simulink model "fullsys_version"  (R2022b)
settings: Solver=VariableStepAuto  StartTime=0.0  StopTime=13  RelTol=1e-3
values from neighbouring files (symbols this model uses):
  alpha_trim = (((Cz_trim + Cz_alp*alpha_0)*(-1*Cm_delm)/Cz_delm) - Cm_0 + (alpha_0*Cm_alpha))/(Cm_alpha + (Cz_alp*(-1*Cm_delm)/Cz_delm))    [variableLoader.m]    (also in variableLoader_OLD.m)
  delt_trim = double(Vin_trim/44.4)    [variableLoader.m]    (also in variableLoader_OLD.m = sqrt((T_trim/(ro*Sprop*Cprop/(2*m))) + velocity*velocity)/kM)
  delta_m_trim = ((alpha_trim - alpha_0)*Cm_alpha + Cm_0)/(-1*Cm_delm)    [variableLoader.m]    (also in variableLoader_OLD.m)
  velocity = 25    [variableLoader.m]    (also in variableLoader_OLD.m)

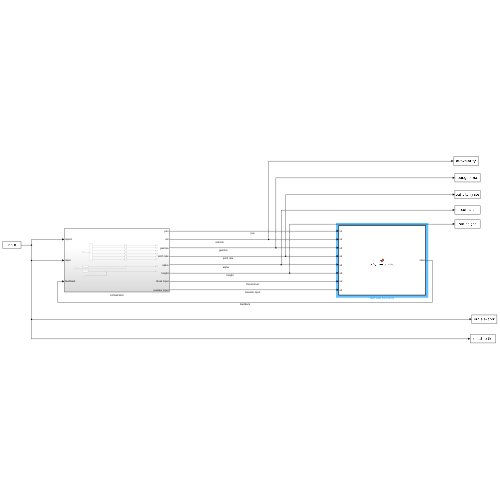
[thumbnail: Simulink's stored preview of the top-level diagram]
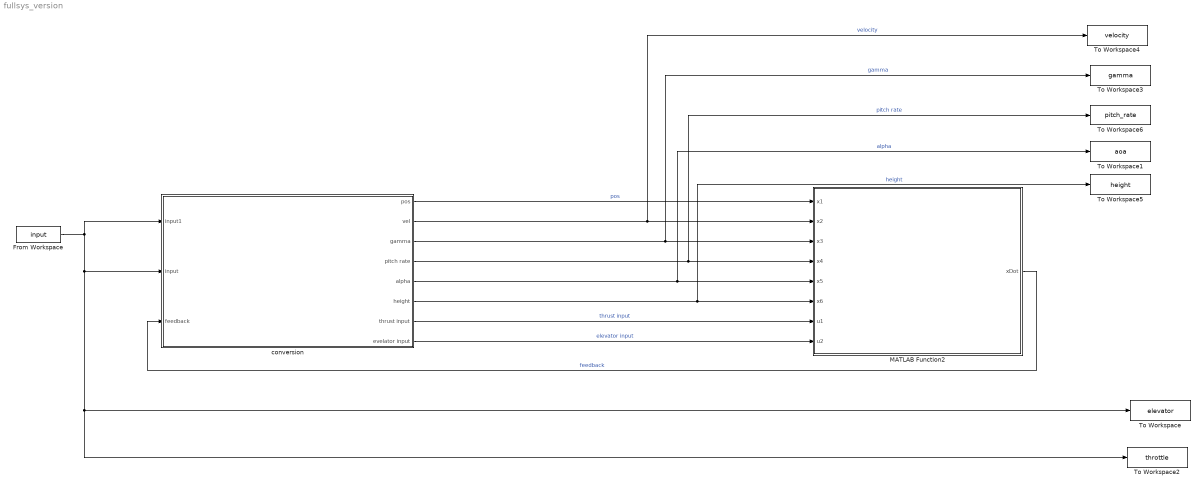
== system fullsys_version ==
  From Workspace : FromWorkspace  VariableName=input  SampleTime=0.02
  MATLAB Function2 : MATLAB Function  TreatAsAtomicUnit=on
  To Workspace : ToWorkspace  VariableName=elevator  SampleTime=0.02
  To Workspace1 : ToWorkspace  VariableName=aoa  SampleTime=0.02
  To Workspace2 : ToWorkspace  VariableName=throttle  SampleTime=0.02
  To Workspace3 : ToWorkspace  VariableName=gamma  SampleTime=0.02
  To Workspace4 : ToWorkspace  VariableName=velocity  SampleTime=0.02
  To Workspace5 : ToWorkspace  VariableName=height  SampleTime=0.02
  To Workspace6 : ToWorkspace  VariableName=pitch_rate  SampleTime=0.02
  conversion : Subsystem
  wires:
  conversion/5(alpha) -> To Workspace1/1, MATLAB Function2/5(x5)  "alpha"
  conversion/2(vel) -> To Workspace4/1, MATLAB Function2/2(x2)  "velocity"
  conversion/1(pos) -> MATLAB Function2/1(x1)  "pos"
  conversion/6(height) -> To Workspace5/1, MATLAB Function2/6(x6)  "height"
  conversion/3(gamma) -> To Workspace3/1, MATLAB Function2/3(x3)  "gamma"
  conversion/7(thrust input) -> MATLAB Function2/7(u1)  "thrust input"
  conversion/8(evelator input) -> MATLAB Function2/8(u2)  "elevator input"
  MATLAB Function2/1(xDot) -> conversion/3(feedback)  "feedback"
  conversion/4(pitch rate) -> To Workspace6/1, MATLAB Function2/4(x4)  "pitch rate"
  From Workspace/1 -> conversion/2(input), To Workspace/1, To Workspace2/1, conversion/1(input1)

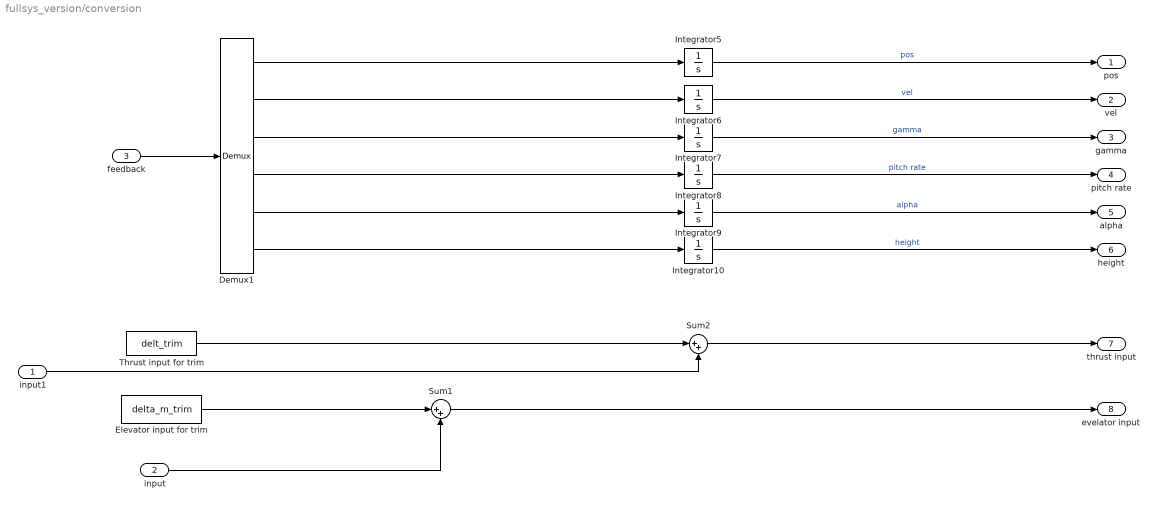
== system fullsys_version/conversion ==
  input1 : Inport
  input : Inport  Port=2
  feedback : Inport  Port=3
  Demux1 : Demux  Outputs=6
  Elevator input for trim : Constant  Value=delta_m_trim  SampleTime=0.02
  Integrator10 : Integrator  InitialCondition=50
  Integrator5 : Integrator
  Integrator6 : Integrator  InitialCondition=velocity
  Integrator7 : Integrator
  Integrator8 : Integrator
  Integrator9 : Integrator  InitialCondition=alpha_trim
  Sum1 : Sum  Inputs=|++
  Sum2 : Sum  Inputs=|++
  Thrust input for trim : Constant  Value=delt_trim  SampleTime=0.02
  pos : Outport
  vel : Outport  Port=2
  gamma : Outport  Port=3
  pitch rate : Outport  Port=4
  alpha : Outport  Port=5
  height : Outport  Port=6
  thrust input : Outport  Port=7
  evelator input : Outport  Port=8
  wires:
  Demux1/4 -> Integrator8/1
  Demux1/3 -> Integrator7/1
  input/1 -> Sum1/2
  Demux1/2 -> Integrator6/1
  Demux1/5 -> Integrator9/1
  Demux1/6 -> Integrator10/1
  Demux1/1 -> Integrator5/1
  Elevator input for trim/1 -> Sum1/1
  Integrator10/1 -> height/1  "height"
  Integrator7/1 -> gamma/1  "gamma"
  Sum1/1 -> evelator input/1
  Integrator9/1 -> alpha/1  "alpha"
  Integrator8/1 -> pitch rate/1  "pitch rate"
  Integrator5/1 -> pos/1  "pos"
  Integrator6/1 -> vel/1  "vel"
  feedback/1 -> Demux1/1
  Thrust input for trim/1 -> Sum2/1
  Sum2/1 -> thrust input/1
  input1/1 -> Sum2/2

== matlab function fullsys_version/MATLAB Function2 ==
function xDot = acDynamics_wind(x1,x2,x3,x4,x5,x6,u1,u2)
    
    Cz_alp = 5.61;
    alpha_0 = -0.04;
    Cz_delm = 0.13;
    Cx_0 = 0.043;
    Cm_0 = 0.0135;
    Cm_alpha = -2.74;
    Cm_q = -38.21;
    L = 0.19;
    Cm_delm = -0.99;
    S = 0.55;
    B = 1.135;
    m = 13.5;
    ro = 1.2682;
    g = 9.8;
    dt = u1;
    delm = u2;

    ki = 0.19/(pi*2.8956*0.1592);
    
    %Thrust model
    KV = 0.0659;
    KQ = 0.0659;
    R = 0.042;
    i0 = 1.5;
    CQ2 = -0.01664;
    CQ1 = 0.00497;
    CQ0 = 0.005230;
    CT2 = -0.1079;
    CT1 = -0.06044;
    CT0 = 0.09357;
    D = 0.5;
    Vin = dt*44.4;

    a = ro*D^5*CQ0/(2*pi)^2;
    b = ro*D^4*CQ1*x2/(2*pi) + KQ*KV/R;
    c = ro*D^3*CQ2*x2*x2 - KQ*Vin/R + KQ*i0;
    np = (-b + sqrt(b*b - 4*a*c))/(2*a);

    T = ro*D^4*CT0*np^2/(4*pi^2) + (ro*D^3*CT1*x2*np/(2*pi)) + ro*D^2*CT2*x2*x2;

    % A/c DYNAMICS
    p = x1;
    V = x2;
    gamma = x3;
    q = x4;
    alpha = x5;
    h = x6;
    
    Cz = Cz_alp*(alpha - alpha_0) + Cz_delm*delm;
    Cx = Cx_0 + ki*Cz^2;
    Cm_G = Cm_0 + Cm_alpha*(alpha - alpha_0) + Cm_q*q*L/V + Cm_delm*delm;
    p_dot = V*cos(gamma); 
    V_dot = (-m*g*sin(gamma) - 0.5*ro*V*V*S*(Cx) + T)/m;
    %V_dot = 0;
    gamma_dot = (m*g*cos(gamma) - 0.5*ro*V*V*S*Cz)/(-m*V);
    
    q_dot = 0.5*ro*V*V*S*L*Cm_G/B;
    
    alpha_dot = q - gamma_dot;
    
    h_dot = V*sin(gamma);
    xDot = [p_dot V_dot gamma_dot q_dot alpha_dot h_dot];
end
